simulink model "SysGenBCM_MR2"  (R2015b)
settings: Solver=ode45  StartTime=0.0  StopTime=2e-3  MaxStep=100e-6  RelTol=1e-3
undefined symbols (not defined in the file): AXI4, Lite
libraries: xbsIndex_r4 x150
(part 2 of 2)

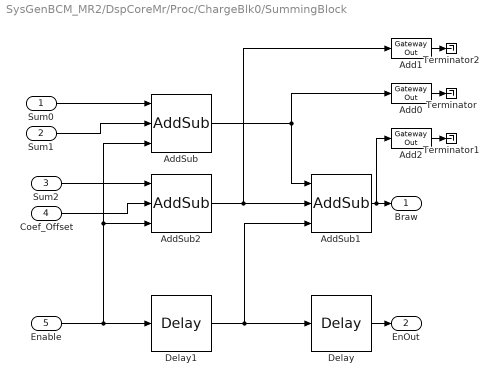
== system SysGenBCM_MR2/DspCoreMr/Proc/ChargeBlk0/SummingBlock ==
  Sum0 : Inport
  Sum1 : Inport  Port=2
  Sum2 : Inport  Port=3
  Coef_Offset : Inport  Port=4
  Enable : Inport  Port=5
  Add0 : xbsIndex_r4/Gateway Out  inherit_from_input=on  hdl_port=on  rows=1  columns=1  UseAsDAC=off  DACChannel='1'  interface=AXI4-Lite  automatic_assignment=off  address_offset=hex2dec('10C')  intf_name=''  intf_description=''  timing_constraint=None  locs_specified=off  LOCs={}  io_standard={}  block_type=gatewayout
  Add1 : xbsIndex_r4/Gateway Out  inherit_from_input=on  hdl_port=on  rows=1  columns=1  UseAsDAC=off  DACChannel='1'  interface=AXI4-Lite  automatic_assignment=off  address_offset=hex2dec('110')  intf_name=''  intf_description=''  timing_constraint=None  locs_specified=off  LOCs={}  io_standard={}  block_type=gatewayout
  Add2 : xbsIndex_r4/Gateway Out  inherit_from_input=on  hdl_port=on  rows=1  columns=1  UseAsDAC=off  DACChannel='1'  interface=AXI4-Lite  automatic_assignment=off  address_offset=hex2dec('114')  intf_name=''  intf_description=''  timing_constraint=None  locs_specified=off  LOCs={}  io_standard={}  block_type=gatewayout
  AddSub : xbsIndex_r4/AddSub  mode=Addition  use_carryin=off  use_carryout=off  en=on  latency=3  precision=Full  arith_type=Unsigned  n_bits=16  bin_pt=14  quantization=Truncate  overflow=Wrap  use_behavioral_HDL=off  hw_selection=Fabric  pipelined=off  dbl_ovrd=off  block_type=addsub
  AddSub1 : xbsIndex_r4/AddSub  mode=Addition  use_carryin=off  use_carryout=off  en=on  latency=3  precision=Full  arith_type=Unsigned  n_bits=16  bin_pt=14  quantization=Truncate  overflow=Wrap  use_behavioral_HDL=off  hw_selection=Fabric  pipelined=off  dbl_ovrd=off  block_type=addsub
  AddSub2 : xbsIndex_r4/AddSub  mode=Addition  use_carryin=off  use_carryout=off  en=on  latency=3  precision=Full  arith_type=Unsigned  n_bits=16  bin_pt=14  quantization=Truncate  overflow=Wrap  use_behavioral_HDL=off  hw_selection=Fabric  pipelined=off  dbl_ovrd=off  block_type=addsub
  Delay : xbsIndex_r4/Delay  rst=off  infoeditControl=Selection of Reset will increase slice count due to use of real FFs and instead of SRLs  en=off  latency=3  reg_retiming=off  dbl_ovrd=off  block_type=delay
      settings: infoedit=Hardware notes: A delay line is a chain, each link of which is an SRL16 or SRL32 followed by a flip-flop.
  Delay1 : xbsIndex_r4/Delay  rst=off  infoeditControl=Selection of Reset will increase slice count due to use of real FFs and instead of SRLs  en=off  latency=3  reg_retiming=off  dbl_ovrd=off  block_type=delay
      settings: infoedit=Hardware notes: A delay line is a chain, each link of which is an SRL16 or SRL32 followed by a flip-flop.
  Terminator : Terminator
  Terminator1 : Terminator
  Terminator2 : Terminator
  Braw : Outport
  EnOut : Outport  Port=2
  wires:
  AddSub/1 -> AddSub1/1, Add0/1
  AddSub1/1 -> Add2/1, Braw/1
  Delay/1 -> EnOut/1
  Enable/1 -> AddSub2/3, AddSub/3, Delay1/1
  Sum1/1 -> AddSub/2
  Sum0/1 -> AddSub/1
  Delay1/1 -> Delay/1, AddSub1/3
  Add0/1 -> Terminator/1
  Add2/1 -> Terminator1/1
  AddSub2/1 -> Add1/1, AddSub1/2
  Sum2/1 -> AddSub2/1
  Coef_Offset/1 -> AddSub2/2
  Add1/1 -> Terminator2/1

== system SysGenBCM_MR2/DspCoreMr/Proc/ChargeBlk1/FloatingConvAndMult0 ==
  Enable : Inport  SampleTime=5.385E-9
  ADCsum0 : Inport  Port=2
  ScoefA : Inport  Port=3  SampleTime=5.385E-9
  Convert0 : xbsIndex_r4/Convert  gui_display_data_type=Fixed-point  arith_type="Signed  (2's comp)"  n_bits=32  bin_pt=0  float_type=Single  exp_bits=8  fraction_bits=24  quantization=Truncate  overflow=Wrap  en=on  latency=1  pipeline=off  dbl_ovrd=off  block_type=convert
  Convert1 : xbsIndex_r4/Convert  gui_display_data_type=Floating-point  arith_type=Floating-point  n_bits=16  bin_pt=14  float_type=Single  exp_bits=8  fraction_bits=24  quantization=Truncate  overflow=Wrap  en=off  latency=1  pipeline=off  dbl_ovrd=off  block_type=convert
  Delay : xbsIndex_r4/Delay  rst=off  infoeditControl=Selection of Reset will increase slice count due to use of real FFs and instead of SRLs  en=off  latency=6  reg_retiming=off  dbl_ovrd=off  block_type=delay
      settings: infoedit=Hardware notes: A delay line is a chain, each link of which is an SRL16 or SRL32 followed by a flip-flop.
  Mult : xbsIndex_r4/Mult  precision=Full  arith_type="Signed  (2's comp)"  n_bits=16  bin_pt=14  quantization=Truncate  overflow=Wrap  en=off  latency=4  use_behavioral_HDL=off  opt=Speed  use_embedded=on  optimum_pipeline=off  pipeline=on  dbl_ovrd=off  use_rpm=on  placement_style=Triangular  block_type=mult
  MultResult : xbsIndex_r4/Gateway Out  inherit_from_input=on  hdl_port=on  rows=1  columns=1  UseAsDAC=off  DACChannel='1'  interface=AXI4-Lite  automatic_assignment=off  address_offset=hex2dec('118')  intf_name=''  intf_description=''  timing_constraint=None  locs_specified=off  LOCs={}  io_standard={}  block_type=gatewayout
  Terminator : Terminator
  ResOut : Outport
  EnOut : Outport  Port=2
  wires:
  Mult/1 -> MultResult/1, ResOut/1
  Convert0/1 -> Convert1/1
  Enable/1 -> Delay/1, Convert0/2
  ScoefA/1 -> Mult/2
  Convert1/1 -> Mult/1
  Delay/1 -> EnOut/1
  ADCsum0/1 -> Convert0/1
  MultResult/1 -> Terminator/1

== system SysGenBCM_MR2/DspCoreMr/Proc/ChargeBlk1/FloatingConvAndMult1 ==
  Enable : Inport  SampleTime=5.385E-9
  ADCsum0 : Inport  Port=2
  ScoefA : Inport  Port=3  SampleTime=5.385E-9
  Convert0 : xbsIndex_r4/Convert  gui_display_data_type=Fixed-point  arith_type="Signed  (2's comp)"  n_bits=32  bin_pt=0  float_type=Single  exp_bits=8  fraction_bits=24  quantization=Truncate  overflow=Wrap  en=on  latency=1  pipeline=off  dbl_ovrd=off  block_type=convert
  Convert1 : xbsIndex_r4/Convert  gui_display_data_type=Floating-point  arith_type=Floating-point  n_bits=16  bin_pt=14  float_type=Single  exp_bits=8  fraction_bits=24  quantization=Truncate  overflow=Wrap  en=off  latency=1  pipeline=off  dbl_ovrd=off  block_type=convert
  Delay : xbsIndex_r4/Delay  rst=off  infoeditControl=Selection of Reset will increase slice count due to use of real FFs and instead of SRLs  en=off  latency=6  reg_retiming=off  dbl_ovrd=off  block_type=delay
      settings: infoedit=Hardware notes: A delay line is a chain, each link of which is an SRL16 or SRL32 followed by a flip-flop.
  Mult : xbsIndex_r4/Mult  precision=Full  arith_type="Signed  (2's comp)"  n_bits=16  bin_pt=14  quantization=Truncate  overflow=Wrap  en=off  latency=4  use_behavioral_HDL=off  opt=Speed  use_embedded=on  optimum_pipeline=off  pipeline=on  dbl_ovrd=off  use_rpm=on  placement_style=Triangular  block_type=mult
  MultResult : xbsIndex_r4/Gateway Out  inherit_from_input=on  hdl_port=on  rows=1  columns=1  UseAsDAC=off  DACChannel='1'  interface=AXI4-Lite  automatic_assignment=off  address_offset=hex2dec('11C')  intf_name=''  intf_description=''  timing_constraint=None  locs_specified=off  LOCs={}  io_standard={}  block_type=gatewayout
  Terminator : Terminator
  ResOut : Outport
  EnOut : Outport  Port=2
  wires:
  Mult/1 -> MultResult/1, ResOut/1
  Convert0/1 -> Convert1/1
  Enable/1 -> Delay/1, Convert0/2
  ScoefA/1 -> Mult/2
  Convert1/1 -> Mult/1
  Delay/1 -> EnOut/1
  ADCsum0/1 -> Convert0/1
  MultResult/1 -> Terminator/1

== system SysGenBCM_MR2/DspCoreMr/Proc/ChargeBlk1/FloatingConvAndMult2 ==
  Enable : Inport  SampleTime=5.385E-9
  ADCsum0 : Inport  Port=2
  ScoefA : Inport  Port=3  SampleTime=5.385E-9
  Convert0 : xbsIndex_r4/Convert  gui_display_data_type=Fixed-point  arith_type="Signed  (2's comp)"  n_bits=32  bin_pt=0  float_type=Single  exp_bits=8  fraction_bits=24  quantization=Truncate  overflow=Wrap  en=on  latency=1  pipeline=off  dbl_ovrd=off  block_type=convert
  Convert1 : xbsIndex_r4/Convert  gui_display_data_type=Floating-point  arith_type=Floating-point  n_bits=16  bin_pt=14  float_type=Single  exp_bits=8  fraction_bits=24  quantization=Truncate  overflow=Wrap  en=off  latency=1  pipeline=off  dbl_ovrd=off  block_type=convert
  Delay : xbsIndex_r4/Delay  rst=off  infoeditControl=Selection of Reset will increase slice count due to use of real FFs and instead of SRLs  en=off  latency=6  reg_retiming=off  dbl_ovrd=off  block_type=delay
      settings: infoedit=Hardware notes: A delay line is a chain, each link of which is an SRL16 or SRL32 followed by a flip-flop.
  Mult : xbsIndex_r4/Mult  precision=Full  arith_type="Signed  (2's comp)"  n_bits=16  bin_pt=14  quantization=Truncate  overflow=Wrap  en=off  latency=4  use_behavioral_HDL=off  opt=Speed  use_embedded=on  optimum_pipeline=off  pipeline=on  dbl_ovrd=off  use_rpm=on  placement_style=Triangular  block_type=mult
  MultResult : xbsIndex_r4/Gateway Out  inherit_from_input=on  hdl_port=on  rows=1  columns=1  UseAsDAC=off  DACChannel='1'  interface=AXI4-Lite  automatic_assignment=off  address_offset=hex2dec('120')  intf_name=''  intf_description=''  timing_constraint=None  locs_specified=off  LOCs={}  io_standard={}  block_type=gatewayout
  Terminator : Terminator
  ResOut : Outport
  EnOut : Outport  Port=2
  wires:
  Mult/1 -> MultResult/1, ResOut/1
  Convert0/1 -> Convert1/1
  Enable/1 -> Delay/1, Convert0/2
  ScoefA/1 -> Mult/2
  Convert1/1 -> Mult/1
  Delay/1 -> EnOut/1
  ADCsum0/1 -> Convert0/1
  MultResult/1 -> Terminator/1

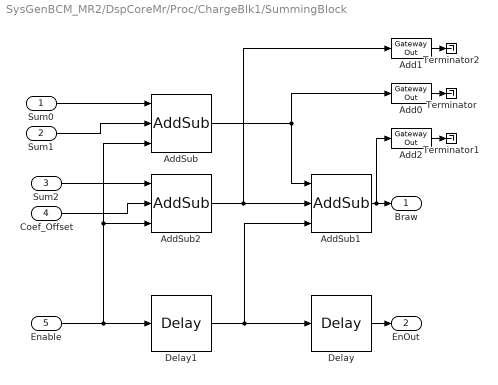
== system SysGenBCM_MR2/DspCoreMr/Proc/ChargeBlk1/SummingBlock ==
  Sum0 : Inport
  Sum1 : Inport  Port=2
  Sum2 : Inport  Port=3
  Coef_Offset : Inport  Port=4
  Enable : Inport  Port=5
  Add0 : xbsIndex_r4/Gateway Out  inherit_from_input=on  hdl_port=on  rows=1  columns=1  UseAsDAC=off  DACChannel='1'  interface=AXI4-Lite  automatic_assignment=off  address_offset=hex2dec('124')  intf_name=''  intf_description=''  timing_constraint=None  locs_specified=off  LOCs={}  io_standard={}  block_type=gatewayout
  Add1 : xbsIndex_r4/Gateway Out  inherit_from_input=on  hdl_port=on  rows=1  columns=1  UseAsDAC=off  DACChannel='1'  interface=AXI4-Lite  automatic_assignment=off  address_offset=hex2dec('128')  intf_name=''  intf_description=''  timing_constraint=None  locs_specified=off  LOCs={}  io_standard={}  block_type=gatewayout
  Add2 : xbsIndex_r4/Gateway Out  inherit_from_input=on  hdl_port=on  rows=1  columns=1  UseAsDAC=off  DACChannel='1'  interface=AXI4-Lite  automatic_assignment=off  address_offset=hex2dec('12C')  intf_name=''  intf_description=''  timing_constraint=None  locs_specified=off  LOCs={}  io_standard={}  block_type=gatewayout
  AddSub : xbsIndex_r4/AddSub  mode=Addition  use_carryin=off  use_carryout=off  en=on  latency=3  precision=Full  arith_type=Unsigned  n_bits=16  bin_pt=14  quantization=Truncate  overflow=Wrap  use_behavioral_HDL=off  hw_selection=Fabric  pipelined=off  dbl_ovrd=off  block_type=addsub
  AddSub1 : xbsIndex_r4/AddSub  mode=Addition  use_carryin=off  use_carryout=off  en=on  latency=3  precision=Full  arith_type=Unsigned  n_bits=16  bin_pt=14  quantization=Truncate  overflow=Wrap  use_behavioral_HDL=off  hw_selection=Fabric  pipelined=off  dbl_ovrd=off  block_type=addsub
  AddSub2 : xbsIndex_r4/AddSub  mode=Addition  use_carryin=off  use_carryout=off  en=on  latency=3  precision=Full  arith_type=Unsigned  n_bits=16  bin_pt=14  quantization=Truncate  overflow=Wrap  use_behavioral_HDL=off  hw_selection=Fabric  pipelined=off  dbl_ovrd=off  block_type=addsub
  Delay : xbsIndex_r4/Delay  rst=off  infoeditControl=Selection of Reset will increase slice count due to use of real FFs and instead of SRLs  en=off  latency=3  reg_retiming=off  dbl_ovrd=off  block_type=delay
      settings: infoedit=Hardware notes: A delay line is a chain, each link of which is an SRL16 or SRL32 followed by a flip-flop.
  Delay1 : xbsIndex_r4/Delay  rst=off  infoeditControl=Selection of Reset will increase slice count due to use of real FFs and instead of SRLs  en=off  latency=3  reg_retiming=off  dbl_ovrd=off  block_type=delay
      settings: infoedit=Hardware notes: A delay line is a chain, each link of which is an SRL16 or SRL32 followed by a flip-flop.
  Terminator : Terminator
  Terminator1 : Terminator
  Terminator2 : Terminator
  Braw : Outport
  EnOut : Outport  Port=2
  wires:
  AddSub/1 -> AddSub1/1, Add0/1
  AddSub1/1 -> Add2/1, Braw/1
  Delay/1 -> EnOut/1
  Enable/1 -> AddSub2/3, AddSub/3, Delay1/1
  Sum1/1 -> AddSub/2
  Sum0/1 -> AddSub/1
  Delay1/1 -> Delay/1, AddSub1/3
  Add0/1 -> Terminator/1
  Add2/1 -> Terminator1/1
  AddSub2/1 -> Add1/1, AddSub1/2
  Sum2/1 -> AddSub2/1
  Coef_Offset/1 -> AddSub2/2
  Add1/1 -> Terminator2/1

== system SysGenBCM_MR2/DspCoreMr/Proc/ChargeBlk2/FloatingConvAndMult0 ==
  Enable : Inport  SampleTime=5.385E-9
  ADCsum0 : Inport  Port=2
  ScoefA : Inport  Port=3  SampleTime=5.385E-9
  Convert0 : xbsIndex_r4/Convert  gui_display_data_type=Fixed-point  arith_type="Signed  (2's comp)"  n_bits=32  bin_pt=0  float_type=Single  exp_bits=8  fraction_bits=24  quantization=Truncate  overflow=Wrap  en=on  latency=1  pipeline=off  dbl_ovrd=off  block_type=convert
  Convert1 : xbsIndex_r4/Convert  gui_display_data_type=Floating-point  arith_type=Floating-point  n_bits=16  bin_pt=14  float_type=Single  exp_bits=8  fraction_bits=24  quantization=Truncate  overflow=Wrap  en=off  latency=1  pipeline=off  dbl_ovrd=off  block_type=convert
  Delay : xbsIndex_r4/Delay  rst=off  infoeditControl=Selection of Reset will increase slice count due to use of real FFs and instead of SRLs  en=off  latency=6  reg_retiming=off  dbl_ovrd=off  block_type=delay
      settings: infoedit=Hardware notes: A delay line is a chain, each link of which is an SRL16 or SRL32 followed by a flip-flop.
  InpSum : xbsIndex_r4/Gateway Out  inherit_from_input=on  hdl_port=on  rows=1  columns=1  UseAsDAC=off  DACChannel='1'  interface=AXI4-Lite  automatic_assignment=off  address_offset=hex2dec('150')  intf_name=''  intf_description=''  timing_constraint=None  locs_specified=off  LOCs={}  io_standard={}  block_type=gatewayout
  Mult : xbsIndex_r4/Mult  precision=Full  arith_type="Signed  (2's comp)"  n_bits=16  bin_pt=14  quantization=Truncate  overflow=Wrap  en=off  latency=4  use_behavioral_HDL=off  opt=Speed  use_embedded=on  optimum_pipeline=off  pipeline=on  dbl_ovrd=off  use_rpm=on  placement_style=Triangular  block_type=mult
  MultResult : xbsIndex_r4/Gateway Out  inherit_from_input=on  hdl_port=on  rows=1  columns=1  UseAsDAC=off  DACChannel='1'  interface=AXI4-Lite  automatic_assignment=off  address_offset=hex2dec('130')  intf_name=''  intf_description=''  timing_constraint=None  locs_specified=off  LOCs={}  io_standard={}  block_type=gatewayout
  Terminator : Terminator
  Terminator1 : Terminator
  ResOut : Outport
  EnOut : Outport  Port=2
  wires:
  Mult/1 -> MultResult/1, ResOut/1
  Convert0/1 -> Convert1/1
  Enable/1 -> Delay/1, Convert0/2
  ScoefA/1 -> Mult/2
  Convert1/1 -> InpSum/1, Mult/1
  Delay/1 -> EnOut/1
  ADCsum0/1 -> Convert0/1
  MultResult/1 -> Terminator/1
  InpSum/1 -> Terminator1/1

== system SysGenBCM_MR2/DspCoreMr/Proc/ChargeBlk2/FloatingConvAndMult1 ==
  Enable : Inport  SampleTime=5.385E-9
  ADCsum0 : Inport  Port=2
  ScoefA : Inport  Port=3  SampleTime=5.385E-9
  Convert0 : xbsIndex_r4/Convert  gui_display_data_type=Fixed-point  arith_type="Signed  (2's comp)"  n_bits=32  bin_pt=0  float_type=Single  exp_bits=8  fraction_bits=24  quantization=Truncate  overflow=Wrap  en=on  latency=1  pipeline=off  dbl_ovrd=off  block_type=convert
  Convert1 : xbsIndex_r4/Convert  gui_display_data_type=Floating-point  arith_type=Floating-point  n_bits=16  bin_pt=14  float_type=Single  exp_bits=8  fraction_bits=24  quantization=Truncate  overflow=Wrap  en=off  latency=1  pipeline=off  dbl_ovrd=off  block_type=convert
  Delay : xbsIndex_r4/Delay  rst=off  infoeditControl=Selection of Reset will increase slice count due to use of real FFs and instead of SRLs  en=off  latency=6  reg_retiming=off  dbl_ovrd=off  block_type=delay
      settings: infoedit=Hardware notes: A delay line is a chain, each link of which is an SRL16 or SRL32 followed by a flip-flop.
  Mult : xbsIndex_r4/Mult  precision=Full  arith_type="Signed  (2's comp)"  n_bits=16  bin_pt=14  quantization=Truncate  overflow=Wrap  en=off  latency=4  use_behavioral_HDL=off  opt=Speed  use_embedded=on  optimum_pipeline=off  pipeline=on  dbl_ovrd=off  use_rpm=on  placement_style=Triangular  block_type=mult
  MultResult : xbsIndex_r4/Gateway Out  inherit_from_input=on  hdl_port=on  rows=1  columns=1  UseAsDAC=off  DACChannel='1'  interface=AXI4-Lite  automatic_assignment=off  address_offset=hex2dec('134')  intf_name=''  intf_description=''  timing_constraint=None  locs_specified=off  LOCs={}  io_standard={}  block_type=gatewayout
  Terminator : Terminator
  ResOut : Outport
  EnOut : Outport  Port=2
  wires:
  Mult/1 -> MultResult/1, ResOut/1
  Convert0/1 -> Convert1/1
  Enable/1 -> Delay/1, Convert0/2
  ScoefA/1 -> Mult/2
  Convert1/1 -> Mult/1
  Delay/1 -> EnOut/1
  ADCsum0/1 -> Convert0/1
  MultResult/1 -> Terminator/1

== system SysGenBCM_MR2/DspCoreMr/Proc/ChargeBlk2/FloatingConvAndMult2 ==
  Enable : Inport  SampleTime=5.385E-9
  ADCsum0 : Inport  Port=2
  ScoefA : Inport  Port=3  SampleTime=5.385E-9
  Convert0 : xbsIndex_r4/Convert  gui_display_data_type=Fixed-point  arith_type="Signed  (2's comp)"  n_bits=32  bin_pt=0  float_type=Single  exp_bits=8  fraction_bits=24  quantization=Truncate  overflow=Wrap  en=on  latency=1  pipeline=off  dbl_ovrd=off  block_type=convert
  Convert1 : xbsIndex_r4/Convert  gui_display_data_type=Floating-point  arith_type=Floating-point  n_bits=16  bin_pt=14  float_type=Single  exp_bits=8  fraction_bits=24  quantization=Truncate  overflow=Wrap  en=off  latency=1  pipeline=off  dbl_ovrd=off  block_type=convert
  Delay : xbsIndex_r4/Delay  rst=off  infoeditControl=Selection of Reset will increase slice count due to use of real FFs and instead of SRLs  en=off  latency=6  reg_retiming=off  dbl_ovrd=off  block_type=delay
      settings: infoedit=Hardware notes: A delay line is a chain, each link of which is an SRL16 or SRL32 followed by a flip-flop.
  Mult : xbsIndex_r4/Mult  precision=Full  arith_type="Signed  (2's comp)"  n_bits=16  bin_pt=14  quantization=Truncate  overflow=Wrap  en=off  latency=4  use_behavioral_HDL=off  opt=Speed  use_embedded=on  optimum_pipeline=off  pipeline=on  dbl_ovrd=off  use_rpm=on  placement_style=Triangular  block_type=mult
  MultResult : xbsIndex_r4/Gateway Out  inherit_from_input=on  hdl_port=on  rows=1  columns=1  UseAsDAC=off  DACChannel='1'  interface=AXI4-Lite  automatic_assignment=off  address_offset=hex2dec('138')  intf_name=''  intf_description=''  timing_constraint=None  locs_specified=off  LOCs={}  io_standard={}  block_type=gatewayout
  Terminator : Terminator
  ResOut : Outport
  EnOut : Outport  Port=2
  wires:
  Mult/1 -> MultResult/1, ResOut/1
  Convert0/1 -> Convert1/1
  Enable/1 -> Delay/1, Convert0/2
  ScoefA/1 -> Mult/2
  Convert1/1 -> Mult/1
  Delay/1 -> EnOut/1
  ADCsum0/1 -> Convert0/1
  MultResult/1 -> Terminator/1

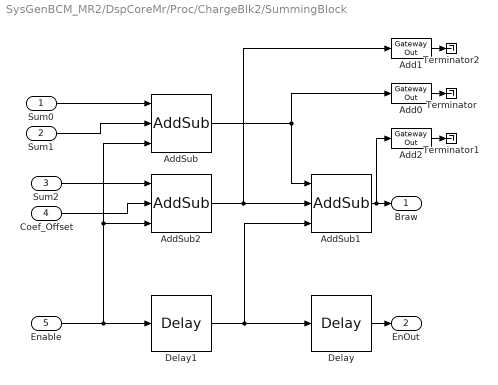
== system SysGenBCM_MR2/DspCoreMr/Proc/ChargeBlk2/SummingBlock ==
  Sum0 : Inport
  Sum1 : Inport  Port=2
  Sum2 : Inport  Port=3
  Coef_Offset : Inport  Port=4
  Enable : Inport  Port=5
  Add0 : xbsIndex_r4/Gateway Out  inherit_from_input=on  hdl_port=on  rows=1  columns=1  UseAsDAC=off  DACChannel='1'  interface=AXI4-Lite  automatic_assignment=off  address_offset=hex2dec('13C')  intf_name=''  intf_description=''  timing_constraint=None  locs_specified=off  LOCs={}  io_standard={}  block_type=gatewayout
  Add1 : xbsIndex_r4/Gateway Out  inherit_from_input=on  hdl_port=on  rows=1  columns=1  UseAsDAC=off  DACChannel='1'  interface=AXI4-Lite  automatic_assignment=off  address_offset=hex2dec('140')  intf_name=''  intf_description=''  timing_constraint=None  locs_specified=off  LOCs={}  io_standard={}  block_type=gatewayout
  Add2 : xbsIndex_r4/Gateway Out  inherit_from_input=on  hdl_port=on  rows=1  columns=1  UseAsDAC=off  DACChannel='1'  interface=AXI4-Lite  automatic_assignment=off  address_offset=hex2dec('144')  intf_name=''  intf_description=''  timing_constraint=None  locs_specified=off  LOCs={}  io_standard={}  block_type=gatewayout
  AddSub : xbsIndex_r4/AddSub  mode=Addition  use_carryin=off  use_carryout=off  en=on  latency=3  precision=Full  arith_type=Unsigned  n_bits=16  bin_pt=14  quantization=Truncate  overflow=Wrap  use_behavioral_HDL=off  hw_selection=Fabric  pipelined=off  dbl_ovrd=off  block_type=addsub
  AddSub1 : xbsIndex_r4/AddSub  mode=Addition  use_carryin=off  use_carryout=off  en=on  latency=3  precision=Full  arith_type=Unsigned  n_bits=16  bin_pt=14  quantization=Truncate  overflow=Wrap  use_behavioral_HDL=off  hw_selection=Fabric  pipelined=off  dbl_ovrd=off  block_type=addsub
  AddSub2 : xbsIndex_r4/AddSub  mode=Addition  use_carryin=off  use_carryout=off  en=on  latency=3  precision=Full  arith_type=Unsigned  n_bits=16  bin_pt=14  quantization=Truncate  overflow=Wrap  use_behavioral_HDL=off  hw_selection=Fabric  pipelined=off  dbl_ovrd=off  block_type=addsub
  Delay : xbsIndex_r4/Delay  rst=off  infoeditControl=Selection of Reset will increase slice count due to use of real FFs and instead of SRLs  en=off  latency=3  reg_retiming=off  dbl_ovrd=off  block_type=delay
      settings: infoedit=Hardware notes: A delay line is a chain, each link of which is an SRL16 or SRL32 followed by a flip-flop.
  Delay1 : xbsIndex_r4/Delay  rst=off  infoeditControl=Selection of Reset will increase slice count due to use of real FFs and instead of SRLs  en=off  latency=3  reg_retiming=off  dbl_ovrd=off  block_type=delay
      settings: infoedit=Hardware notes: A delay line is a chain, each link of which is an SRL16 or SRL32 followed by a flip-flop.
  Terminator : Terminator
  Terminator1 : Terminator
  Terminator2 : Terminator
  Braw : Outport
  EnOut : Outport  Port=2
  wires:
  AddSub/1 -> AddSub1/1, Add0/1
  AddSub1/1 -> Add2/1, Braw/1
  Delay/1 -> EnOut/1
  Enable/1 -> AddSub2/3, AddSub/3, Delay1/1
  Sum1/1 -> AddSub/2
  Sum0/1 -> AddSub/1
  Delay1/1 -> Delay/1, AddSub1/3
  Add0/1 -> Terminator/1
  Add2/1 -> Terminator1/1
  AddSub2/1 -> Add1/1, AddSub1/2
  Sum2/1 -> AddSub2/1
  Coef_Offset/1 -> AddSub2/2
  Add1/1 -> Terminator2/1
